simulink model "PrviIDrugiZad"  (R2016b)
settings: Solver=VariableStepAuto  StartTime=-50  StopTime=50  RelTol=1e-3
libraries: simulink x7
settings Model: Creator=Luka  LastModifiedBy=Luka

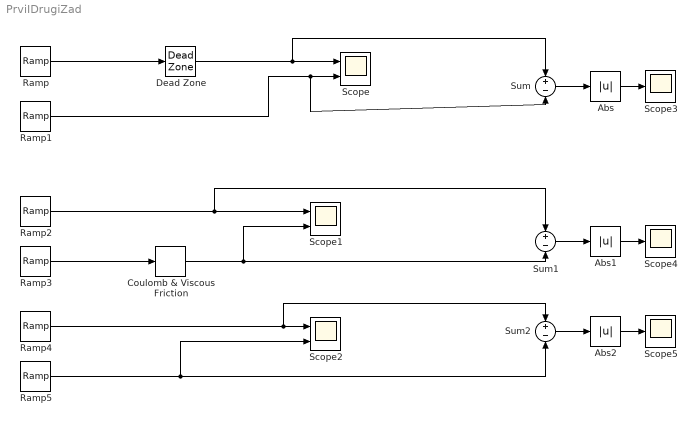
== system PrviIDrugiZad ==
  Abs : Abs
  Abs1 : Abs
  Abs2 : Abs
  Coulomb & Viscous Friction : simulink/Discontinuities/Coulomb & Viscous Friction  offset=2  gain=0.8
  Dead Zone : DeadZone  LowerValue=0  UpperValue=5/6  SaturateOnIntegerOverflow=on
  Ramp : simulink/Sources/Ramp  slope=5/24  start=-50  X0=-10
  Ramp{1..4} (4 alike) : simulink/Sources/Ramp  slope=1/5  start=-50  X0=-10
  Ramp5 : simulink/Sources/Ramp  slope=4/25  start=-50  X0=-6
  Scope : Scope  NumInputPorts=2
  Scope1 : Scope  NumInputPorts=2
  Scope2 : Scope  NumInputPorts=2
  Scope3 : Scope
  Scope4 : Scope
  Scope5 : Scope
  Sum : Sum  Inputs=+-
  Sum1 : Sum  Inputs=+-
  Sum2 : Sum  Inputs=+-
  wires:
  Ramp1/1 -> Sum/2, Scope/2
  Ramp/1 -> Dead Zone/1
  Dead Zone/1 -> Sum/1, Scope/1
  Coulomb & Viscous Friction/1 -> Scope1/2, Sum1/2
  Ramp2/1 -> Sum1/1, Scope1/1
  Ramp3/1 -> Coulomb & Viscous Friction/1
  Ramp4/1 -> Sum2/1, Scope2/1
  Ramp5/1 -> Sum2/2, Scope2/2
  Sum/1 -> Abs/1
  Abs/1 -> Scope3/1
  Abs1/1 -> Scope4/1
  Sum1/1 -> Abs1/1
  Abs2/1 -> Scope5/1
  Sum2/1 -> Abs2/1
